simulink model "sil_test"  (R2022b)
settings: Solver=VariableStepAuto  StartTime=0.0  StopTime=inf  RelTol=1e-3
undefined symbols (not defined in the file): battery_monitor, battery_monitor_lib, BM_STATUSES, canChannel, DI_STATUSES, driver_interface, driver_interface_lib, Ended, governor, governor_lib, MI_STATUSES, motor_interface, motor_interface_lib, simp_vd_interface, simp_vd_lib, Single
libraries: canmsglib x16, canlib x10, simulink x6, speedgoatlib_IO191 x5, slrealtimeiplib x3, AMK_comms_plant_lib x1, BMS_plant_lib x1, speedgoatlib_IO614 x1, slrealtimeutilitieslib x1, etargetslib x1
(part 3 of 3)

== system sil_test/driver_interface/potentiometerProcessing4 ==
  FractionIn : Inport
  Interval Test Dynamic : simulink/Logic and Bit Operations/Interval Test Dynamic  IntervalClosedRight=on  IntervalClosedLeft=on  OutDataTypeStr=boolean
  LowerPotentiometerLimit1 : Constant  Value=0  OutDataTypeStr=double
  NOT : Logic  Operator=NOT  IconShape=distinctive  AllPortsSameDT=off  OutDataTypeStr=boolean
  UpperPotentiometerLimit1 : Constant  OutDataTypeStr=double
  FractionOut : Outport
  FractionError : Outport  Port=2
  wires:
  NOT/1 -> FractionError/1
  FractionIn/1 -> FractionOut/1, Interval Test Dynamic/2
  Interval Test Dynamic/1 -> NOT/1  "withinNominalRange"
  UpperPotentiometerLimit1/1 -> Interval Test Dynamic/1
  LowerPotentiometerLimit1/1 -> Interval Test Dynamic/3

== system sil_test/simp_vd_interface/Running Avg ==
  note: Change number of samples to compute average from
  Raw_Torque : Inport
  Divide : Product  Inputs=*/
  Sum of Elements : Sum  Inputs=+
  Tapped Delay : simulink/Discrete/Tapped Delay  vinit=0  samptime=-1  NumDelays=10  DelayOrder=Oldest  includeCurrent=off
  Vector Concatenate : Concatenate
  Width : Width
  Running_Avg : Outport
  wires:
  Divide/1 -> Running_Avg/1
  Vector Concatenate/1 -> Width/1, Sum of Elements/1
  Raw_Torque/1 -> Vector Concatenate/1, Tapped Delay/1
  Width/1 -> Divide/2
  Tapped Delay/1 -> Vector Concatenate/2
  Sum of Elements/1 -> Divide/1

== system sil_test/simp_vd_interface/TC ==
  note: SR = V_driven/V_idle - 1
  Idle_wheel_spd : Inport
  Driven_wheel_spd : Inport  Port=2
  Target_slip : Inport  Port=3
  Constant : Constant
  Divide : Product  Inputs=*/
  Set lower bound to 0 : Saturate  UpperLimit=inf  LowerLimit=0
  Subtract : Sum  Inputs=+-
  vd_tc : Stateflow chart  TreatAsAtomicUnit=on
  TC_scale_factor : Outport
  wires:
  Set lower bound to 0/1 -> vd_tc/1(Actual_slip)
  Constant/1 -> Subtract/2
  Divide/1 -> Subtract/1
  Driven_wheel_spd/1 -> Divide/1
  Idle_wheel_spd/1 -> Divide/2
  Target_slip/1 -> vd_tc/2(Target_slip)  "Desired slip = 0.2"
  Subtract/1 -> Set lower bound to 0/1  "Actual_slip"
  vd_tc/1(TC_scale_factor) -> TC_scale_factor/1

== stateflow chart sil_test/simp_vd_interface/TC/vd_tc ==
  state TC_off
    en, du:
    TC_scale_factor = 1;
  state TC_on
    en, du:
    TC_scale_factor = 0.5;
  state TC_on1
    en, du:
    TC_scale_factor = 0.25;
  state TC_on2
    en, du:
    TC_scale_factor = 0;
  (default) -> TC_off
  TC_off -> TC_on2 : [after(50,msec) && Actual_slip > Target_slip]
  TC_on -> TC_off : after(33,msec)
  TC_on1 -> TC_on : after(33,msec)
  TC_on2 -> TC_on1 : [after(33,msec) && Actual_slip <= Target_slip]
  data: Actual_slip input; Target_slip input; TC_scale_factor output

== stateflow chart sil_test/driver_interface/driver_interface ==
  state INIT
    en:
    GOV_e_diSts = DI_STATUSES.DI_STS_INIT;
    b_ReadyToDrive=false;
    DI_b_driverSpeaker = false;
  state DI_running
    state Waiting_for_driver
      en:
      GOV_e_diSts = ...
      DI_STATUSES.WAITING_FOR_DRVR;
    state Driver_requested_start
      en:
      GOV_e_diSts =...
      DI_STATUSES.HV_START_REQ;
    state Motor_start_request
      en:
      GOV_e_diSts = ...
      DI_STATUSES.READY_TO_DRIVE_REQ;
    state Ready_to_drive
      en:
      b_ReadyToDrive = true;
      GOV_e_diSts = DI_RUNNING;
      state SpeakerOn_
        en:
        DI_b_driverSpeaker = true;
      state SpeakerOff
        en:
        DI_b_driverSpeaker = false;
      (default) -> SpeakerOn_
      SpeakerOn_ -> SpeakerOff : after(2,sec)
    Waiting_for_driver -> Driver_requested_start : [(DI_b_DriverButton==1)]
    Driver_requested_start -> Motor_start_request : [GOV_e_diCmd == DI_CMD.HV_ON && DI_b_DriverButton == 1]
    Motor_start_request -> Ready_to_drive : [GOV_e_diCmd ==...
        |  DI_CMD.READY_TO_DRIVE  && (p_brakePedalPos>0.1)]
  state DI_error
    en:
    GOV_e_diSts = DI_STATUSES.DI_ERROR;
  state Vehicle_coasting
    en:
    b_ReadyToDrive = false;
    GOV_e_diSts = DI_STATUSES.DI_IDLE;
  (default) -> INIT
  Ready_to_drive -> INIT [order 2] : [GOV_e_diCmd == DI_SHUTDOWN]
  INIT -> Waiting_for_driver : [GOV_e_diCmd == DI_CMD.DI_CMD_INIT]
  DI_running -> DI_error : [b_DriverInterfaceError==1]
  Ready_to_drive -> Vehicle_coasting [order 1] : [GOV_e_diCmd ==...
      |  DI_CMD.RUN_ERROR]
  data: GOV_e_diCmd input Enum: DI_CMD; DI_b_DriverButton input; GOV_e_diSts output Enum: DI_STATUSES size=1; b_DriverInterfaceError input; DI_b_driverSpeaker output boolean; b_ReadyToDrive output boolean; p_brakePedalPos input

== stateflow chart sil_test/simp_vd_interface/vd_screenshot_check ==
  state Run
    en, du:
    DI_p_motorTorqueRequest = DI_p_driverTorqueRequest;
  state Stop
    en, du:
    DI_p_motorTorqueRequest = 0;
  (default) -> Run
  Run -> Stop : [DI_p_driverTorqueRequest >= 0.25 && brake_on]
  Stop -> Run : [DI_p_driverTorqueRequest < 0.05 && ~brake_on]
  data: DI_p_driverTorqueRequest input; brake_on input; DI_p_motorTorqueRequest output

== stateflow chart sil_test/battery_monitor/battery_monitor ==
  state InitialState
    entry:
    GOV_e_bmSts = ...
    BM_STATUSES.BM_INIT;
  state StartupSuperstate
    state StartupState1
      entry:
      GOV_e_bmSts = BM_STATUSES.BM_IDLE;
    state StartupState
      entry:
      GOV_e_bmSts = BM_STATUSES.BM_STARTUP;
    state InitializePrechargeState
      entry:
      GOV_e_bmSts = BM_STATUSES.INIT_PRECHARGE;
    state PrechargeState
      entry:
      GOV_e_bmSts = BM_STATUSES.PRECHARGE;
    state RunningState
      entry:
      GOV_e_bmSts = BM_STATUSES.BM_RUNNING;
    StartupState1 -> StartupState : [BM_b_prechrgContactorSts == 0 && BM_b_HVnegContactorSts == 1 && BM_b_HVposContactorSts == 0]
    StartupState -> InitializePrechargeState : [BM_b_prechrgContactorSts == 1 && BM_b_HVnegContactorSts == 1 && BM_b_HVposContactorSts == 0]
    InitializePrechargeState -> PrechargeState : [BM_b_prechrgContactorSts == 1 && BM_b_HVnegContactorSts == 1 && BM_b_HVposContactorSts == 1]
    PrechargeState -> RunningState : [BM_b_prechrgContactorSts == 0 && BM_b_HVnegContactorSts == 1 && BM_b_HVposContactorSts == 1]
    RunningState -> RunningState : [BM_b_prechrgContactorSts == 0 && BM_b_HVnegContactorSts == 1 && BM_b_HVposContactorSts == 1]
  state InterruptState
    %Lost HVIL during startup or running
    en:
    GOV_e_bmSts = ...
    BM_STATUSES.HVIL_INTERRUPT;
  state LowSoC
    %HV battery low
    en:
    GOV_e_bmSts = ...
    BM_STATUSES.BM_LOW_SOC;
  (default) -> InitialState
  InterruptState -> InitialState : after(5,sec)[BM_HvilFeedback == 1]
  InitialState -> StartupState1 : [BM_b_prechrgContactorSts == 0 &&...
      |  BM_b_HVnegContactorSts == 0 &&...
      |  BM_b_HVposContactorSts == 0 &&...
      |  GOV_e_bmCmd == BM_CMD.HV_STARTUP &&...
      |  BM_HvilFeedback == 1]
  StartupSuperstate -> InterruptState [order 1] : [BM_HvilFeedback == 0]
  StartupSuperstate -> LowSoC [order 2] : [BM_PackSOC < 30]
  data: GOV_e_bmCmd input; BM_b_prechrgContactorSts input; BM_b_HVposContactorSts input; BM_b_HVnegContactorSts input; GOV_e_bmSts output Enum: BM_STATUSES; BM_HvilFeedback input; BM_PackSOC input

== stateflow chart sil_test/battery_monitor/bm_control ==
  state StartupCMD
    en:
    BM_b_prechargeContactorCMD = 0;
    BM_b_HVnegContactorCMD = 0;
    BM_b_HVposContactorCMD = 0;
  state StartupSuperstate
    state Close_HVneg1
      en:
      BM_b_prechargeContactorCMD = 0;
      BM_b_HVnegContactorCMD = 1;
      BM_b_HVposContactorCMD = 0;
    state Close_precharge
      en:
      BM_b_prechargeContactorCMD = 1;
      BM_b_HVnegContactorCMD = 1;
      BM_b_HVposContactorCMD = 0;
    state Close_HVpos
      en:
      BM_b_prechargeContactorCMD = 1;
      BM_b_HVnegContactorCMD = 1;
      BM_b_HVposContactorCMD = 1;
    state Open_precharge
      en, du:
      BM_b_prechargeContactorCMD = 0;
      BM_b_HVnegContactorCMD = 1;
      BM_b_HVposContactorCMD = 1;
    Close_HVneg1 -> Close_precharge : after(100,msec)[GOV_e_bmSts == BM_STATUSES.BM_STARTUP]
    Close_precharge -> Close_HVpos : after(6500,msec)[GOV_e_bmSts == BM_STATUSES.INIT_PRECHARGE]
    Close_HVpos -> Open_precharge : after(100,msec)[GOV_e_bmSts == BM_STATUSES.PRECHARGE]
    Open_precharge -> Open_precharge : [GOV_e_bmSts == BM_STATUSES.BM_RUNNING]
  (default) -> StartupCMD
  StartupSuperstate -> StartupCMD : [GOV_e_bmSts == BM_STATUSES.HVIL_INTERRUPT || ...
      | GOV_e_bmSts == BM_STATUSES.BM_LOW_SOC]
  StartupCMD -> Close_HVneg1 : [GOV_e_bmSts == BM_STATUSES.BM_IDLE]
  data: BM_b_prechargeContactorCMD output; BM_b_HVposContactorCMD output; BM_b_HVnegContactorCMD output; GOV_e_bmSts input

== matlab function sil_test/simp_vd_interface/avg ==
  data: wspdLF input; Idle_wheel_spd output; wspdRF input
function Idle_wheel_spd = fcn(wspdLF,wspdRF)
Idle_wheel_spd = (wspdLF+wspdRF)/2;

== matlab function sil_test/simp_vd_interface/return greater ==
  data: wspdLR input; Driven_wheel_spd output; wspdRR input
function Driven_wheel_spd = fcn(wspdLR,wspdRR)
if wspdLR > wspdRR
    Driven_wheel_spd = wspdLR;
else
    Driven_wheel_spd = wspdRR;
end

== stateflow chart sil_test/governor/governer_stateflow ==
  state Initialize_outputs
    en:
    GOV_e_govSts = GOV_STATUSES.GOV_INIT;
    GOV_e_diCmd = DI_CMD.DI_CMD_INIT;
    motorStartCount = 0;
  state STARTUP
    en:
    GOV_e_govSts = GOV_STATUSES.GOV_STARTUP;
    state HV_startup
      en:
      GOV_e_bmCmd = ...
      BM_CMD.HV_STARTUP;
    state ReadyToDrive
      en:
      GOV_e_diCmd = ...
      DI_CMD.HV_ON;
    state Command_motor_startup
      en:
      GOV_e_miCmd = MI_CMD.CMD_STARTUP;
      motorStartCount = motorStartCount+1;
    state Send_ReadyToDrive
      en:
      GOV_e_diCmd = DI_CMD.READY_TO_DRIVE;
    (default) -> HV_startup
    HV_startup -> ReadyToDrive : [GOV_e_bmSts == BM_STATUSES.BM_RUNNING]
    ReadyToDrive -> Command_motor_startup : [GOV_e_diSts == DI_STATUSES.READY_TO_DRIVE_REQ]
    Command_motor_startup -> Send_ReadyToDrive : [GOV_e_miSts == ...
        | MI_STATUSES.RUNNING]
  state STARTUP_ERROR
    state HV_startup_error
      en:
      GOV_e_govSts =...
      GOV_STATUSES.HV_STARTUP_ERROR;
    state Err_reset
      during:
      GOV_e_miCmd=...
      MI_CMD.ERR_RESET;
    state Motor_faulted
      en:
      % tell other motor to shutdown
      % if still running
      GOV_e_miCmd=...
      MI_CMD.CMD_SHUTDOWN;
      GOV_e_govSts =...
      GOV_STATUSES.MOTOR_STARTUP_ERROR;
    state DriverInterface_Error
      en:
      GOV_e_govSts =...
      GOV_STATUSES.GOV_DI_ERROR;
    (junction 88) -> Err_reset [order 2]
    (junction 88) -> Motor_faulted [order 1] : [motorStartCount >= 5]
  state Vehicle_shutdown
    en:
    GOV_e_govSts = GOV_STATUSES.GOV_SHUTDOWN;
    GOV_e_miCmd = MI_CMD.CMD_SHUTDOWN;
    GOV_e_diCmd = DI_CMD.DI_SHUTDOWN;
  state RUNNING_ERROR
    state HV_run_error
      en:
      GOV_e_diCmd = ...
      DI_CMD.RUN_ERROR;
      GOV_e_govSts =...
      GOV_STATUSES.HV_RUN_ERROR;
    state Motor_run_error
      en:
      GOV_e_diCmd = ...
      DI_CMD.RUN_ERROR;
      GOV_e_govSts =...
      GOV_STATUSES.MOTOR_RUN_ERROR;
  state RUNNING
    en:
    GOV_e_govSts = GOV_STATUSES.GOV_RUNNING;
  (default) -> Initialize_outputs
  HV_startup_error -> Initialize_outputs : [GOV_e_bmSts == BM_STATUSES.BM_INIT]
  Vehicle_shutdown -> Initialize_outputs : [GOV_e_bmSts == BM_STATUSES.BM_INIT]
  Initialize_outputs -> HV_startup : after(2,sec)[GOV_e_diSts == ...
      | DI_STATUSES.HV_START_REQ]
  STARTUP -> HV_startup_error [order 1] : [GOV_e_bmSts == ...
      | BM_STATUSES.HVIL_INTERRUPT]
  Err_reset -> STARTUP : [GOV_e_miSts ==...
      |  MI_STATUSES.OFF]
  STARTUP -> (junction 88) [order 3] : [GOV_e_miSts == ...
      | MI_STATUSES.MI_STS_ERROR]
  RUNNING -> Vehicle_shutdown [order 1] : [GOV_e_bmSts == BM_STATUSES.HVIL_INTERRUPT || ...
      | GOV_e_bmSts == BM_STATUSES.BM_LOW_SOC]
  STARTUP -> DriverInterface_Error [order 2] : [GOV_e_diSts ==...
      | DI_STATUSES.DI_ERROR]
  Send_ReadyToDrive -> RUNNING : [GOV_e_diSts == ...
      | DI_STATUSES.DI_RUNNING]
  RUNNING -> HV_run_error [order 2] : [GOV_e_bmSts == ...
      | BM_STATUSES.ERR_RUNNING]
  RUNNING -> Motor_run_error [order 3] : [GOV_e_miSts == ...
      | MI_STATUSES.MI_STS_ERROR]
  data: GOV_e_bmSts input; GOV_e_vdSts input; GOV_e_miSts input; GOV_e_diSts input; GOV_e_bmCmd output size=1; GOV_e_vdCmd output uint8 size=1; GOV_e_miCmd output Enum: MI_CMD size=1; GOV_e_diCmd output Enum: DI_CMD size=1; motorStartCount local uint16; GOV_e_govSts output

== stateflow chart sil_test/motor_interface/mi_left ==
  state motorOff_waitingForGov
    en:
    MI_motorStatus = MI_STATUSES.OFF;
    AMK_bInverterOn_tx = 0;
    AMK_bDcOn_tx = 0;
    AMK_bEnable = 0;
    AMK_bErrorReset = 0;
    AMK_TargetVelocity = 0;
    AMK_TorqueLimitPositiv = 0;
    AMK_TorqueLimitNegativ = 0;
    MI_InverterEn = 0;
  state AMK_startup
    state waiting_sysReady
      en:
      MI_motorStatus = MI_STATUSES.STARTUP;
    state toggleDCon
      en:
      AMK_bDcOn_tx = 1;
    state enforceSetpointsZero
      en:
      AMK_TargetVelocity = 0;
      AMK_TorqueLimitPositiv = 0;
      AMK_TorqueLimitNegativ = 0;
    state commandOn
      en:
      AMK_bEnable = 1;
      AMK_bInverterOn_tx = 1;
    waiting_sysReady -> (junction 67) [order 2] : [AMK_bError==1]
    waiting_sysReady -> toggleDCon [order 1] : [AMK_bSystemReady==1]
    toggleDCon -> (junction 67) [order 2] : [AMK_bError==1]
    toggleDCon -> AMK_startup.enforceSetpointsZero [order 1] : [(AMK_bDcOn_rx==1) ...
        | && (AMK_bQuitDcOn==1)]
    AMK_startup.enforceSetpointsZero -> (junction 67) [order 2] : [AMK_bError==1]
    commandOn -> (junction 67) [order 2] : [AMK_bError==1]
    AMK_startup.enforceSetpointsZero -> commandOn [order 1] : after(100,msec)
  state AMK_errorReset
    state toggleReset
      en:
      AMK_bErrorReset = 0;
    state sendReset
      en:
      AMK_bErrorReset = 1;
    state toggleEnable
      en:
      AMK_bEnable = 0;
    state enforceSetpointsZero
      en:
      AMK_TargetVelocity = 0;
      AMK_TorqueLimitPositiv = 0;
      AMK_TorqueLimitNegativ = 0;
      AMK_bInverterOn_tx = 0;
    sendReset -> toggleReset : after(500,msec)
    toggleEnable -> sendReset : after(500,msec)
    AMK_errorReset.enforceSetpointsZero -> toggleEnable : [AMK_bInverterOn_rx==0]
  state AMK_shutdown
    en:
    AMK_TargetVelocity = 0;
    AMK_TorqueLimitPositiv = 0;
    AMK_TorqueLimitNegativ = 0;
    MI_InverterEn = 0;
  state AMK_errorDetected
    en:
    MI_motorStatus = MI_STATUSES.MI_STS_ERROR;
  state AMK_ready
    en, du:
    MI_motorStatus = MI_STATUSES.READY;
    MI_InverterEn = 1;
  state AMK_running
    during:
    MI_motorStatus = MI_STATUSES.RUNNING;
    AMK_TargetVelocity = VD_T_motorSpeedRequest;
    AMK_TorqueLimitPositiv = VD_T_motorTorqueLimitPositive;
    AMK_TorqueLimitNegativ = VD_T_motorTorqueLimitNegative;
  toggleReset -> motorOff_waitingForGov : [AMK_bSystemReady==1]
  commandOn -> AMK_ready [order 1] : [AMK_bInverterOn_rx ==1]
  motorOff_waitingForGov -> waiting_sysReady : [GOV_e_miCmd == MI_CMD.CMD_STARTUP]
  (default) -> motorOff_waitingForGov
  (junction 67) -> AMK_errorDetected
  AMK_shutdown -> motorOff_waitingForGov : after(500,msec)
  AMK_running -> AMK_shutdown [order 2] : [GOV_e_miCmd == MI_CMD.CMD_SHUTDOWN]
  AMK_errorDetected -> AMK_errorReset.enforceSetpointsZero : [GOV_e_miCmd == MI_CMD.ERR_RESET]
  AMK_ready -> AMK_errorDetected [order 1] : [AMK_bError==1]
  AMK_running -> AMK_errorDetected [order 1] : [AMK_bError==1]
  AMK_ready -> AMK_running [order 2] : [(AMK_bQuitInverterOn == 1) && ...
      | (AMK_bError == 0)]
  data: GOV_e_miCmd input Enum: MI_CMD; AMK_bReserve input; AMK_ActualVelocity input; AMK_MagnetizingCurrent input; AMK_TorqueCurrent input; AMK_bDcOn_rx input; AMK_bDerating input; AMK_bError input; AMK_bInverterOn_rx input; AMK_bQuitDcOn input; AMK_bQuitInverterOn input; MI_motorStatus output Enum: MI_STATUSES size=1; AMK_bSystemReady input; AMK_bWarn input; AMK_ErrorInfo input; AMK_TempIGBT input; AMK_TempInverter input; AMK_TempMotor input; VD_T_motorSpeedRequest input; AMK_bInverterOn_tx output uint8 size=1; AMK_bDcOn_tx output uint8 size=1; AMK_bEnable output uint8 size=1; AMK_bErrorReset output uint8 size=1; AMK_TargetVelocity output single size=1; AMK_TorqueLimitPositiv output single size=1; AMK_TorqueLimitNegativ output single size=1; VD_T_motorTorqueLimitPositive input; VD_T_motorTorqueLimitNegative input; MI_InverterEn output

== stateflow chart sil_test/motor_interface/mi_right ==
  state motorOff_waitingForGov
    en:
    MI_motorStatus = MI_STATUSES.OFF;
    AMK_bInverterOn_tx = 0;
    AMK_bDcOn_tx = 0;
    AMK_bEnable = 0;
    AMK_bErrorReset = 0;
    AMK_TargetVelocity = 0;
    AMK_TorqueLimitPositiv = 0;
    AMK_TorqueLimitNegativ = 0;
    MI_InverterEn = 0;
  state AMK_startup
    state waiting_sysReady
      en:
      MI_motorStatus = MI_STATUSES.STARTUP;
    state toggleDCon
      en:
      AMK_bDcOn_tx = 1;
    state enforceSetpointsZero
      en:
      AMK_TargetVelocity = 0;
      AMK_TorqueLimitPositiv = 0;
      AMK_TorqueLimitNegativ = 0;
    state commandOn
      en:
      AMK_bEnable = 1;
      AMK_bInverterOn_tx = 1;
    waiting_sysReady -> (junction 67) [order 2] : [AMK_bError==1]
    waiting_sysReady -> toggleDCon [order 1] : [AMK_bSystemReady==1]
    toggleDCon -> (junction 67) [order 2] : [AMK_bError==1]
    toggleDCon -> AMK_startup.enforceSetpointsZero [order 1] : [(AMK_bDcOn_rx==1) ...
        | && (AMK_bQuitDcOn==1)]
    AMK_startup.enforceSetpointsZero -> (junction 67) [order 2] : [AMK_bError==1]
    commandOn -> (junction 67) [order 2] : [AMK_bError==1]
    AMK_startup.enforceSetpointsZero -> commandOn [order 1] : after(100,msec)
  state AMK_errorReset
    state toggleReset
      en:
      AMK_bErrorReset = 0;
    state sendReset
      en:
      AMK_bErrorReset = 1;
    state toggleEnable
      en:
      AMK_bEnable = 0;
    state enforceSetpointsZero
      en:
      AMK_TargetVelocity = 0;
      AMK_TorqueLimitPositiv = 0;
      AMK_TorqueLimitNegativ = 0;
      AMK_bInverterOn_tx = 0;
    sendReset -> toggleReset : after(500,msec)
    toggleEnable -> sendReset : after(500,msec)
    AMK_errorReset.enforceSetpointsZero -> toggleEnable : [AMK_bInverterOn_rx==0]
  state AMK_shutdown
    en:
    AMK_TargetVelocity = 0;
    AMK_TorqueLimitPositiv = 0;
    AMK_TorqueLimitNegativ = 0;
    MI_InverterEn = 0;
  state AMK_errorDetected
    en:
    MI_motorStatus = MI_STATUSES.MI_STS_ERROR;
  state AMK_ready
    en, du:
    MI_motorStatus = MI_STATUSES.READY;
    MI_InverterEn = 1;
  state AMK_running
    during:
    MI_motorStatus = MI_STATUSES.RUNNING;
    AMK_TargetVelocity = VD_T_motorSpeedRequest;
    AMK_TorqueLimitPositiv = VD_T_motorTorqueLimitPositive;
    AMK_TorqueLimitNegativ = VD_T_motorTorqueLimitNegative;
  toggleReset -> motorOff_waitingForGov : [AMK_bSystemReady==1]
  commandOn -> AMK_ready [order 1] : [AMK_bInverterOn_rx ==1]
  motorOff_waitingForGov -> waiting_sysReady : [GOV_e_miCmd == MI_CMD.CMD_STARTUP]
  (default) -> motorOff_waitingForGov
  (junction 67) -> AMK_errorDetected
  AMK_shutdown -> motorOff_waitingForGov : after(500,msec)
  AMK_running -> AMK_shutdown [order 2] : [GOV_e_miCmd == MI_CMD.CMD_SHUTDOWN]
  AMK_errorDetected -> AMK_errorReset.enforceSetpointsZero : [GOV_e_miCmd == MI_CMD.ERR_RESET]
  AMK_ready -> AMK_errorDetected [order 1] : [AMK_bError==1]
  AMK_running -> AMK_errorDetected [order 1] : [AMK_bError==1]
  AMK_ready -> AMK_running [order 2] : [(AMK_bQuitInverterOn == 1) && ...
      | (AMK_bError == 0)]
  data: GOV_e_miCmd input Enum: MI_CMD; AMK_bReserve input; AMK_ActualVelocity input; AMK_MagnetizingCurrent input; AMK_TorqueCurrent input; AMK_bDcOn_rx input; AMK_bDerating input; AMK_bError input; AMK_bInverterOn_rx input; AMK_bQuitDcOn input; AMK_bQuitInverterOn input; MI_motorStatus output Enum: MI_STATUSES size=1; AMK_bSystemReady input; AMK_bWarn input; AMK_ErrorInfo input; AMK_TempIGBT input; AMK_TempInverter input; AMK_TempMotor input; VD_T_motorSpeedRequest input; AMK_bInverterOn_tx output uint8 size=1; AMK_bDcOn_tx output uint8 size=1; AMK_bEnable output uint8 size=1; AMK_bErrorReset output uint8 size=1; AMK_TargetVelocity output single size=1; AMK_TorqueLimitPositiv output single size=1; AMK_TorqueLimitNegativ output single size=1; VD_T_motorTorqueLimitPositive input; VD_T_motorTorqueLimitNegative input; MI_InverterEn output
